simulink model "inverted_pendulum_parameter_estimation"  (R2025a)
settings: Solver=FixedStepAuto  StartTime=0.0  StopTime=10.0  FixedStep=0.0001  MaxStep=0.001  RelTol=1e-3
values from neighbouring files (symbols this model uses):
  p_btheta = 0.00372326875104    [parameters.mat]
  p_bx = 2.60549125077    [parameters.mat]
  p_G = 6.6666    [parameters.mat]
  p_g = 9.81    [parameters.mat]
  p_Iw = 0.00013229942248    [parameters.mat]
  p_Jp = 0.00022725    [parameters.mat]
  p_Ke = 0.0492216052224    [parameters.mat]
  p_Kt = 0.0213162134254    [parameters.mat]
  p_l = 0.15    [parameters.mat]
  p_La = 0.00290272767215    [parameters.mat]
  p_M = 0.698    [parameters.mat]
  p_m = 0.0303    [parameters.mat]
  p_r = 0.0255    [parameters.mat]
  p_Ra = 31.0735233211    [parameters.mat]
undefined symbols (not defined in the file or in its folder): p_Dz
settings Model: Creator=nopla  LastModifiedBy=nopla
settings DataIOCC: SaveFormat=StructureWithTime  OutputOption=AdditionalOutputTimes  OutputTimes=SDO_OutputTimes  ReturnWorkspaceOutputsName=SDOSimTest_Log

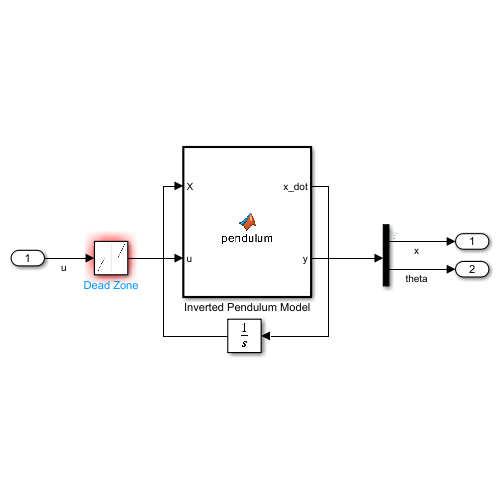
[thumbnail: Simulink's stored preview of the top-level diagram]
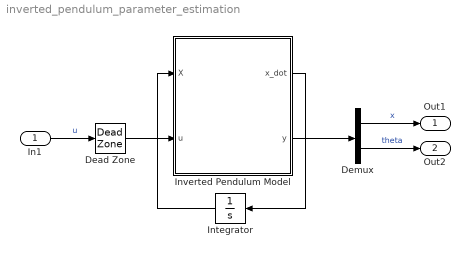
== system inverted_pendulum_parameter_estimation ==
  In1 : Inport
  Dead Zone : DeadZone  LowerValue=-p_Dz  UpperValue=p_Dz
  Demux : Demux  Outputs=2
  Integrator : Integrator  InitialCondition=[0; 0; 0; 0; 0]
  Inverted Pendulum Model : MATLAB Function  TreatAsAtomicUnit=on
  Out1 : Outport
  Out2 : Outport  Port=2
  wires:
  Inverted Pendulum Model/1(x_dot) -> Integrator/1
  Integrator/1 -> Inverted Pendulum Model/1(X)
  Inverted Pendulum Model/2(y) -> Demux/1
  In1/1 -> Dead Zone/1  "u"
  Demux/1 -> Out1/1  "x"
  Demux/2 -> Out2/1  "theta"
  Dead Zone/1 -> Inverted Pendulum Model/2(u)

== matlab function inverted_pendulum_parameter_estimation/Inverted Pendulum Model ==
  data: x_dot output size=[5 1]; y output; X input size=[5 1]; u input; p_M parameter; p_m parameter; p_g parameter; p_l parameter; p_r parameter; p_Iw parameter; p_G parameter; p_Jp parameter; p_bx parameter; p_btheta parameter; p_Kt parameter; p_Ke parameter; p_Ra parameter; p_La parameter
function [x_dot, y] = pendulum(X, u, p_M, p_m, p_g, p_l, p_r, p_Iw, p_G, p_Jp, p_bx, p_btheta, p_Kt, p_Ke, p_Ra, p_La)
% 台車型倒立振子の状態空間動力学
% 
% 入力:
%   X: 状態ベクトル [x; x_dot; theta; theta_dot; i] (5x1)
%   u: 入力電圧 V (スカラー)
%   params: パラメータ構造体

params = [p_M; p_m; p_g; p_l; p_r; p_Iw; p_G; p_Jp; p_bx; p_btheta; p_Kt; p_Ke; p_Ra; p_La];

x_dot = nonlinear_dynamics(X, u, params);

y = [X(1); X(3)];

end
